simulink library "util_orbit_dynamics_lib"  (R2015b)
settings: Solver=VariableStepAuto  StartTime=0.0  StopTime=10.0  RelTol=1e-3
undefined symbols (not defined in the file or in its folder): central_body_gravity_mu, dt_perigee, ecc_anom, mean_anom, true_anom
libraries: util_orbit_dynamics_lib x15, util_common_lib x8, simulink_extras x2
settings Model: Creator=Mark Agbayani  LastModifiedBy=Mark Agbayani

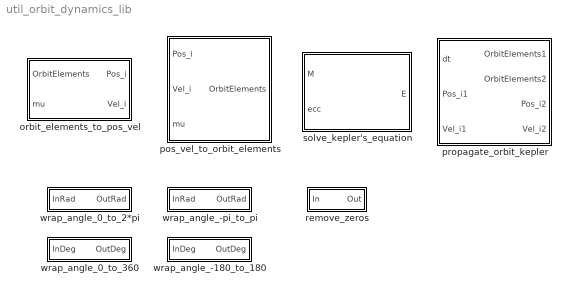
== system util_orbit_dynamics_lib ==
  orbit_elements_to_pos_vel : Subsystem
  pos_vel_to_orbit_elements : Subsystem
  propagate_orbit_kepler : Subsystem
  remove_zeros : Subsystem
  solve_kepler's_equation : Subsystem
  wrap_angle_-180_to_180 : Subsystem
      mask Display:
      | text(.5,.5,'-180< ang <+180', ...
      | 	'HorizontalAlignment','Center',...
      | 	'VerticalAlignment','middle')
  wrap_angle_-pi_to_pi : Subsystem
      mask Display:
      | text(.5,.5,'-pi < ang < +pi', ...
      | 	'HorizontalAlignment','Center',...
      | 	'VerticalAlignment','middle')
  wrap_angle_0_to_2*pi : Subsystem
      mask Display:
      | text(0.5,0.5,'0 < ang < 2*pi', ...
      | 	'HorizontalAlignment','Center',...
      | 	'VerticalAlignment','middle')
  wrap_angle_0_to_360 : Subsystem
      mask Display:
      | text(0.5,0.5,'0 < ang < 360', ...
      | 	'HorizontalAlignment','Center',...
      | 	'VerticalAlignment','middle')

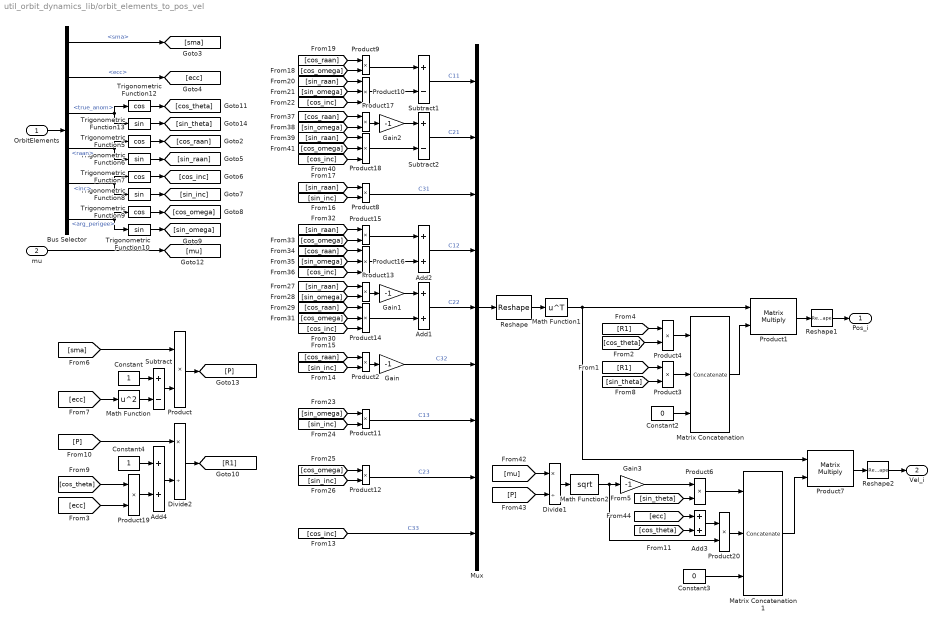
== system util_orbit_dynamics_lib/orbit_elements_to_pos_vel ==
  OrbitElements : Inport
  mu : Inport  Port=2
  Add{1..4} (4 alike) : Sum
  Bus Selector : BusSelector  OutputSignals=sma,ecc,true_anom,raan,inc,arg_perigee
  Constant : Constant
  Constant2 : Constant  Value=0
  Constant3 : Constant  Value=0
  Constant4 : Constant
  Divide1 : Product  Inputs=*/
  Divide2 : Product  Inputs=*/
  Gain{,1..3} (4 alike) : Gain  Gain=-1
  Math Function : Math  Operator=square  SaturateOnIntegerOverflow=on
  Math Function1 : Math  Operator=transpose  SaturateOnIntegerOverflow=on
  Math Function2 : Math  Operator=sqrt  SaturateOnIntegerOverflow=on
  Matrix Concatenation : Concatenate  NumInputs=3  Mode=Multidimensional array
  Matrix Concatenation1 : Concatenate  NumInputs=3  Mode=Multidimensional array
  Mux : Mux  Inputs=9
  Product{,2..4,6,8..9,11..13,15,17,19..20} (14 alike) : Product  RndMeth=Zero
  Product1 : Product  Multiplication=Matrix(*)  RndMeth=Zero
  Product{10,14,16,18} (4 alike) : Product  Inputs=3  RndMeth=Zero
  Product7 : Product  Multiplication=Matrix(*)  RndMeth=Zero
  Reshape : Reshape  OutputDimensionality=Customize  OutputDimensions=[3,3]
  Reshape1 : Reshape
  Reshape2 : Reshape
  Subtract : Sum  Inputs=+-
  Subtract1 : Sum  Inputs=+-
  Subtract2 : Sum  Inputs=+-
  Trigonometric Function{6,8,10,13} (4 alike) : Trigonometry
  Trigonometric Function{5,7,9,12} (4 alike) : Trigonometry  Operator=cos
  Pos_i : Outport
  Vel_i : Outport  Port=2
  wires:
  Matrix Concatenation1/1 -> Product7/2
  mu/1 -> [mu]
  [ecc] -> Math Function/1
  Constant/1 -> Subtract/1
  Math Function/1 -> Subtract/2
  Subtract/1 -> Product/2
  [sma] -> Product/1
  Product/1 -> [P]
  [R1] -> Product4/1
  [cos_theta] -> Product4/2
  Product4/1 -> Matrix Concatenation/1
  Product3/1 -> Matrix Concatenation/2
  Constant2/1 -> Matrix Concatenation/3
  Product6/1 -> Matrix Concatenation1/1
  Constant3/1 -> Matrix Concatenation1/3
  Mux/1 -> Reshape/1
  Reshape/1 -> Math Function1/1
  Trigonometric Function5/1 -> [cos_raan]
  Trigonometric Function6/1 -> [sin_raan]
  Trigonometric Function7/1 -> [cos_inc]
  Trigonometric Function8/1 -> [sin_inc]
  Trigonometric Function9/1 -> [cos_omega]
  Trigonometric Function10/1 -> [sin_omega]
  [cos_inc] -> Mux/9  "C33"
  Gain/1 -> Mux/6  "C32"
  Product2/1 -> Gain/1
  [cos_raan] -> Product2/1
  [sin_inc] -> Product2/2
  [sin_raan] -> Product8/1
  [sin_inc] -> Product8/2
  Product8/1 -> Mux/3  "C31"
  Subtract1/1 -> Mux/1  "C11"
  [cos_raan] -> Product9/1
  [cos_omega] -> Product9/2
  Product9/1 -> Subtract1/1
  Product10/1 -> Subtract1/2
  [sin_raan] -> Product10/1
  [sin_omega] -> Product10/2
  [cos_inc] -> Product10/3
  Product11/1 -> Mux/7  "C13"
  [sin_omega] -> Product11/1
  [sin_inc] -> Product11/2
  Math Function1/1 -> Product1/1, Product7/1
  [cos_omega] -> Product12/1
  [sin_inc] -> Product12/2
  Product12/1 -> Mux/8  "C23"
  [sin_raan] -> Product13/1
  [sin_omega] -> Product13/2
  Product13/1 -> Gain1/1
  Gain1/1 -> Add1/1
  [cos_raan] -> Product14/1
  [cos_omega] -> Product14/2
  [cos_inc] -> Product14/3
  Product14/1 -> Add1/2
  Add1/1 -> Mux/5  "C22"
  Subtract2/1 -> Mux/2  "C21"
  Add2/1 -> Mux/4  "C12"
  [sin_raan] -> Product15/1
  [cos_omega] -> Product15/2
  Product15/1 -> Add2/1
  Product16/1 -> Add2/2
  [cos_raan] -> Product16/1
  [sin_omega] -> Product16/2
  [cos_inc] -> Product16/3
  [cos_raan] -> Product17/1
  [sin_omega] -> Product17/2
  Product17/1 -> Gain2/1
  Gain2/1 -> Subtract2/1
  [sin_raan] -> Product18/1
  [cos_omega] -> Product18/2
  [cos_inc] -> Product18/3
  Product18/1 -> Subtract2/2
  [mu] -> Divide1/1
  [P] -> Divide1/2
  Divide1/1 -> Math Function2/1
  Math Function2/1 -> Gain3/1, Product20/2
  [sin_theta] -> Product6/2
  [cos_theta] -> Add3/2
  Gain3/1 -> Product6/1
  [ecc] -> Add3/1
  Add3/1 -> Product20/1
  Product20/1 -> Matrix Concatenation1/2
  Matrix Concatenation/1 -> Product1/2
  [P] -> Divide2/1
  Add4/1 -> Divide2/2
  Constant4/1 -> Add4/1
  [cos_theta] -> Product19/1
  Product19/1 -> Add4/2
  [ecc] -> Product19/2
  Divide2/1 -> [R1]
  Trigonometric Function12/1 -> [cos_theta]
  Trigonometric Function13/1 -> [sin_theta]
  [R1] -> Product3/1
  [sin_theta] -> Product3/2
  OrbitElements/1 -> Bus Selector/1
  Bus Selector/1 -> [sma]  "<sma>"
  Bus Selector/2 -> [ecc]  "<ecc>"
  Bus Selector/3 -> Trigonometric Function12/1, Trigonometric Function13/1  "<true_anom>"
  Bus Selector/4 -> Trigonometric Function5/1, Trigonometric Function6/1  "<raan>"
  Bus Selector/5 -> Trigonometric Function8/1, Trigonometric Function7/1  "<inc>"
  Bus Selector/6 -> Trigonometric Function9/1, Trigonometric Function10/1  "<arg_perigee>"
  Product1/1 -> Reshape1/1
  Product7/1 -> Reshape2/1
  Reshape1/1 -> Pos_i/1
  Reshape2/1 -> Vel_i/1

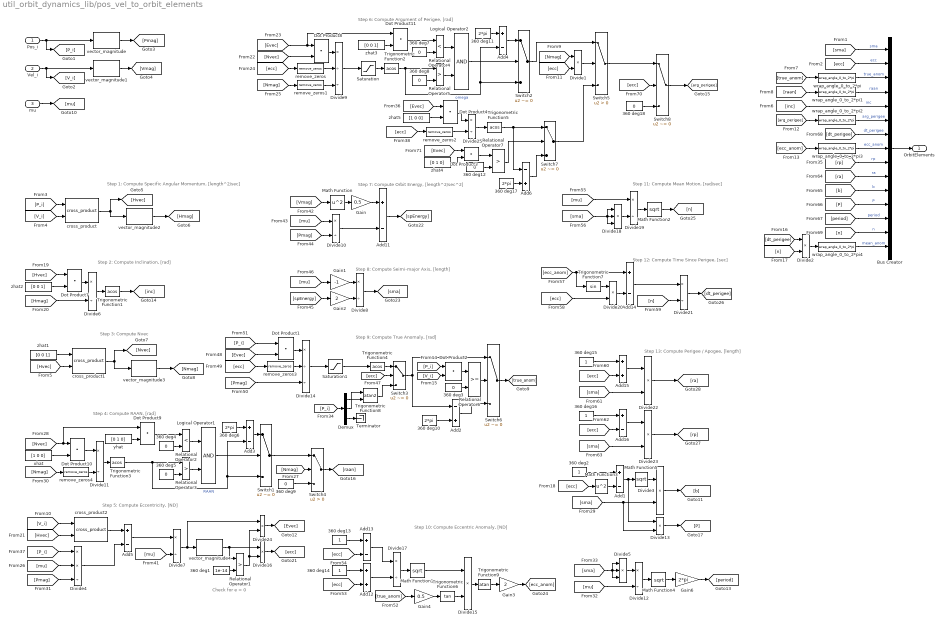
== system util_orbit_dynamics_lib/pos_vel_to_orbit_elements ==
  note: Step 1: Compute Specific Angular Momentum, [length^2/sec]
  note: Step 2: Compute Inclination, [rad]
  note: Step 3: Compute Nvec
  note: Step 4: Compute RAAN, [rad]
  note: Step 5: Compute Eccentricity, [ND]
  note: Step 6: Compute Argument of Perigee, [rad]
  note: Step 7: Compute Orbit Energy, [length^2/sec^2]
  note: Step 8: Compute Seimi-major Axis, [length]
  note: Step 9: Compute True Anomaly, [rad]
  note: Step 10: Compute Eccentric Anomaly, [ND]
  note: Step 11: Compute Mean Motion, [rad/sec]
  note: Step 12: Compute Time Since Perigee, [sec]
  note: Step 13: Compute Perigee / Apogee, [length]
  note: Check for e = 0
  Pos_i : Inport
  Vel_i : Inport  Port=2
  mu : Inport  Port=3
  360 deg1 : Constant  Value=1e-14
  360 deg{6,10..11,17} (4 alike) : Constant  Value=2*pi
  360 deg{3..5,7..9,12,18} (8 alike) : Constant  Value=0
  360 deg{2,13..16} (5 alike) : Constant
  Add{1,3..5,11,13..14,16} (8 alike) : Sum  Inputs=+-
  Add12 : Sum
  Add15 : Sum
  Add2 : Sum  Inputs=-+
  Add6 : Sum  Inputs=-+
  Bus Creator : BusCreator  Inputs=15
  Demux : Demux  Outputs=3
  Divide{1..3,13,15..16,20,22..24} (10 alike) : Product  Inputs=**
  Divide{6..8,10..12,17,19,21,25} (10 alike) : Product  Inputs=*/
  Divide14 : Product  Inputs=*//
  Divide18 : Product  Inputs=***
  Divide4 : Product  Inputs=**/
  Divide5 : Product  Inputs=***
  Divide9 : Product  Inputs=*//
  Dot Product{1..4,7..11} (9 alike) : DotProduct  InputSameDT=on  OutDataTypeStr=Inherit: Inherit via internal rule
  Gain : Gain  Gain=0.5
  Gain1 : Gain  Gain=-1
  Gain2 : Gain  Gain=2
  Gain3 : Gain  Gain=2
  Gain4 : Gain  Gain=0.5
  Gain6 : Gain  Gain=2*pi
  Logical Operator1 : Logic  AllPortsSameDT=off  OutDataTypeStr=float('double')
  Logical Operator2 : Logic  AllPortsSameDT=off  OutDataTypeStr=float('double')
  Math Function : Math  Operator=square  SaturateOnIntegerOverflow=on
  Math Function{1..2,4..5} (4 alike) : Math  Operator=sqrt  SaturateOnIntegerOverflow=on
  Math Function3 : Math  Operator=square  SaturateOnIntegerOverflow=on
  Relational Operator1 : RelationalOperator  Operator=>  OutDataTypeStr=float('double')
  Relational Operator2 : RelationalOperator  Operator=<  OutDataTypeStr=boolean
  Relational Operator3 : RelationalOperator  Operator=>  OutDataTypeStr=boolean
  Relational Operator4 : RelationalOperator  Operator=<  OutDataTypeStr=boolean
  Relational Operator5 : RelationalOperator  Operator=>  OutDataTypeStr=boolean
  Relational Operator6 : RelationalOperator  OutDataTypeStr=float('double')
  Relational Operator7 : RelationalOperator  Operator=>  OutDataTypeStr=float('double')
  Saturation : Saturate  UpperLimit=1  LowerLimit=-1
  Saturation1 : Saturate  UpperLimit=1  LowerLimit=-1
  Switch{1..3,6..8} (6 alike) : Switch  Criteria=u2 ~= 0
  Switch4 : Switch  Criteria=u2 > Threshold
  Switch5 : Switch  Criteria=u2 > Threshold
  Terminator : Terminator
  Trigonometric Function{1..5} (5 alike) : Trigonometry  Operator=acos
  Trigonometric Function6 : Trigonometry  Operator=tan
  Trigonometric Function7 : Trigonometry
  Trigonometric Function8 : Trigonometry  Operator=atan2
  Trigonometric Function9 : Trigonometry  Operator=atan
  cross_product : util_common_lib/cross_product  SystemSampleTime=-1
  cross_product1 : util_common_lib/cross_product  SystemSampleTime=-1
  cross_product2 : util_common_lib/cross_product  SystemSampleTime=-1
  remove_zeros{,1..4} (5 alike) : util_orbit_dynamics_lib/remove_zeros  SystemSampleTime=-1
  vector_magnitude{,1..4} (5 alike) : util_common_lib/vector_magnitude  SystemSampleTime=-1
  wrap_angle_0_to_2*pi{,1..4} (5 alike) : util_orbit_dynamics_lib/wrap_angle_0_to_2*pi  SystemSampleTime=-1
  xhat : Constant  Value=[1 0 0]
  yhat : Constant  Value=[0 1 0]
  zhat1 : Constant  Value=[0 0 1]
  zhat2 : Constant  Value=[0 0 1]
  zhat3 : Constant  Value=[0 0 1]
  zhat4 : Constant  Value=[0 1 0]
  zhat5 : Constant  Value=[1 0 0]
  OrbitElements : Outport
  wires:
  wrap_angle_0_to_2*pi4/1 -> Bus Creator/15  "mean_anom"
  [n] -> Bus Creator/14  "n"
  [period] -> Bus Creator/13  "period"
  [P] -> Bus Creator/12  "P"
  [b] -> Bus Creator/11  "b"
  [ra] -> Bus Creator/10  "ra"
  [rp] -> Bus Creator/9  "rp"
  wrap_angle_0_to_2*pi3/1 -> Bus Creator/8  "ecc_anom"
  [dt_perigee] -> Bus Creator/7  "dt_perigee"
  [sma] -> Divide23/2
  [ecc] -> Add16/2
  Add16/1 -> Divide23/1
  360 deg16/1 -> Add16/1
  [sma] -> Divide22/2
  [ecc] -> Add15/2
  Add15/1 -> Divide22/1
  360 deg15/1 -> Add15/1
  Divide21/1 -> [dt_perigee]
  [n] -> Divide21/2
  Add14/1 -> Divide21/1
  Divide20/1 -> Add14/2
  [ecc] -> Divide20/2
  Trigonometric Function7/1 -> Divide20/1
  [ecc_anom] -> Trigonometric Function7/1, Add14/1
  Math Function2/1 -> [n]
  Divide19/1 -> Math Function2/1
  [sma] -> Divide18/3, Divide18/2, Divide18/1
  Divide18/1 -> Divide19/2
  [mu] -> Divide19/1
  Add12/1 -> Divide17/2
  Add13/1 -> Divide17/1
  [ecc] -> Add13/2
  360 deg13/1 -> Add13/1
  [ecc] -> Add12/2
  360 deg14/1 -> Add12/1
  Divide17/1 -> Math Function1/1
  Gain4/1 -> Trigonometric Function6/1
  [true_anom] -> Gain4/1
  Trigonometric Function6/1 -> Divide15/2
  Math Function1/1 -> Divide15/1
  Divide15/1 -> Trigonometric Function9/1
  Gain3/1 -> [ecc_anom]
  Dot Product1/1 -> Divide14/1
  [Pmag] -> Divide14/3
  [Evec] -> Dot Product1/2
  [P_i] -> Dot Product1/1
  Trigonometric Function4/1 -> Switch3/1
  [ecc] -> Switch3/2
  Divide8/1 -> [sma]
  Gain1/1 -> Divide8/1
  Gain2/1 -> Divide8/2
  [spEnergy] -> Gain2/1
  [mu] -> Gain1/1
  Add11/1 -> [spEnergy]
  Math Function/1 -> Gain/1
  Gain/1 -> Add11/1
  Divide10/1 -> Add11/2
  [Pmag] -> Divide10/2
  [mu] -> Divide10/1
  [Vmag] -> Math Function/1
  vector_magnitude4/1 -> Relational Operator1/1, Divide16/1
  Divide7/1 -> vector_magnitude4/1, Divide24/1
  [mu] -> Divide7/2
  Add5/1 -> Divide7/1
  Divide4/1 -> Add5/2
  [Pmag] -> Divide4/3
  [mu] -> Divide4/2
  [P_i] -> Divide4/1
  [Hvec] -> cross_product2/2
  [V_i] -> cross_product2/1
  cross_product2/1 -> Add5/1
  Dot Product9/1 -> Relational Operator2/1
  Add3/1 -> Switch1/1
  Logical Operator1/1 -> Switch1/2
  360 deg6/1 -> Add3/1
  Relational Operator3/1 -> Logical Operator1/2
  Relational Operator2/1 -> Logical Operator1/1
  360 deg5/1 -> Relational Operator3/2
  360 deg4/1 -> Relational Operator2/2
  yhat/1 -> Dot Product9/2
  Bus Creator/1 -> OrbitElements/1
  wrap_angle_0_to_2*pi2/1 -> Bus Creator/6  "arg_perigee"
  [inc] -> Bus Creator/5  "inc"
  wrap_angle_0_to_2*pi1/1 -> Bus Creator/4  "raan"
  wrap_angle_0_to_2*pi/1 -> Bus Creator/3  "true_anom"
  [ecc] -> Bus Creator/2  "ecc"
  [sma] -> Bus Creator/1  "sma"
  [Nvec] -> Dot Product9/1, Dot Product10/1
  [Nmag] -> remove_zeros4/1
  Trigonometric Function3/1 -> Switch1/3, Add3/2, Relational Operator3/1  "RAAN"
  Divide11/1 -> Trigonometric Function3/1
  Dot Product10/1 -> Divide11/1
  xhat/1 -> Dot Product10/2
  Divide6/1 -> Trigonometric Function1/1
  Trigonometric Function1/1 -> [inc]
  Dot Product7/1 -> Divide6/1
  [Hmag] -> Divide6/2
  [Hvec] -> Dot Product7/1
  zhat2/1 -> Dot Product7/2
  zhat1/1 -> cross_product1/1
  [Hvec] -> cross_product1/2
  cross_product1/1 -> vector_magnitude3/1, [Nvec]
  vector_magnitude3/1 -> [Nmag]
  cross_product/1 -> vector_magnitude2/1, [Hvec]
  vector_magnitude2/1 -> [Hmag]
  [V_i] -> cross_product/2
  [P_i] -> cross_product/1
  Vel_i/1 -> vector_magnitude1/1, [V_i]
  vector_magnitude/1 -> [Pmag]
  vector_magnitude1/1 -> [Vmag]
  Pos_i/1 -> vector_magnitude/1, [P_i]
  [true_anom] -> wrap_angle_0_to_2*pi/1
  [raan] -> wrap_angle_0_to_2*pi1/1
  [arg_perigee] -> wrap_angle_0_to_2*pi2/1
  [ecc_anom] -> wrap_angle_0_to_2*pi3/1
  mu/1 -> [mu]
  [Nmag] -> Switch4/2
  360 deg9/1 -> Switch4/3
  Switch4/1 -> [raan]
  Switch1/1 -> Switch4/1
  Divide14/1 -> Saturation1/1
  [Evec] -> Dot Product11/1, Dot Product8/1
  Dot Product11/1 -> Relational Operator4/1
  Add4/1 -> Switch2/1
  Logical Operator2/1 -> Switch2/2
  360 deg11/1 -> Add4/1
  Relational Operator5/1 -> Logical Operator2/2
  Relational Operator4/1 -> Logical Operator2/1
  360 deg8/1 -> Relational Operator5/2
  360 deg7/1 -> Relational Operator4/2
  zhat3/1 -> Dot Product11/2
  Trigonometric Function2/1 -> Switch2/3, Add4/2, Relational Operator5/1  "omega"
  Divide9/1 -> Saturation/1
  Dot Product8/1 -> Divide9/1
  [Nmag] -> remove_zeros1/1
  [ecc] -> remove_zeros/1
  [Nvec] -> Dot Product8/2
  [Nmag] -> Divide1/1
  [ecc] -> Divide1/2
  Divide1/1 -> Switch5/2
  Switch2/1 -> Switch5/1
  Switch6/1 -> [true_anom]
  Switch3/1 -> Switch6/1, Add2/1
  [P_i] -> Dot Product2/1
  [V_i] -> Dot Product2/2
  [dt_perigee] -> Divide2/1
  [n] -> Divide2/2
  Divide2/1 -> wrap_angle_0_to_2*pi4/1
  [sma] -> Divide3/2, Divide13/2
  [ecc] -> Math Function3/1
  Add1/1 -> Math Function5/1, Divide13/1
  360 deg2/1 -> Add1/1
  Math Function3/1 -> Add1/2
  Divide3/1 -> [b]
  Divide12/1 -> Math Function4/1
  [sma] -> Divide5/2, Divide5/3, Divide5/1
  Divide5/1 -> Divide12/1
  [mu] -> Divide12/2
  Math Function4/1 -> Gain6/1
  Gain6/1 -> [period]
  Math Function5/1 -> Divide3/1
  Divide13/1 -> [P]
  Divide23/1 -> [rp]
  Divide22/1 -> [ra]
  [P_i] -> Demux/1
  Demux/3 -> Terminator/1
  Demux/1 -> Trigonometric Function8/2
  Demux/2 -> Trigonometric Function8/1
  Trigonometric Function8/1 -> Switch3/3
  360 deg1/1 -> Relational Operator1/2
  Relational Operator1/1 -> Divide16/2, Divide24/2
  Divide16/1 -> [ecc]
  Divide24/1 -> [Evec]
  Dot Product2/1 -> Relational Operator6/1
  360 deg3/1 -> Relational Operator6/2
  Relational Operator6/1 -> Switch6/2
  remove_zeros1/1 -> Divide9/3
  remove_zeros/1 -> Divide9/2
  remove_zeros4/1 -> Divide11/2
  Trigonometric Function9/1 -> Gain3/1
  zhat5/1 -> Dot Product4/2
  [Evec] -> Dot Product4/1
  Dot Product4/1 -> Divide25/1
  [ecc] -> remove_zeros2/1
  remove_zeros2/1 -> Divide25/2
  Divide25/1 -> Trigonometric Function5/1
  [ecc] -> remove_zeros3/1
  remove_zeros3/1 -> Divide14/2
  360 deg10/1 -> Add2/2
  Add2/1 -> Switch6/3
  Saturation1/1 -> Trigonometric Function4/1
  Saturation/1 -> Trigonometric Function2/1
  Trigonometric Function5/1 -> Switch7/1, Add6/1
  360 deg12/1 -> Relational Operator7/2
  Dot Product3/1 -> Relational Operator7/1
  Relational Operator7/1 -> Switch7/2
  360 deg17/1 -> Add6/2
  Add6/1 -> Switch7/3
  Switch7/1 -> Switch5/3
  zhat4/1 -> Dot Product3/2
  [Evec] -> Dot Product3/1
  Switch5/1 -> Switch8/1
  [ecc] -> Switch8/2
  360 deg18/1 -> Switch8/3
  Switch8/1 -> [arg_perigee]

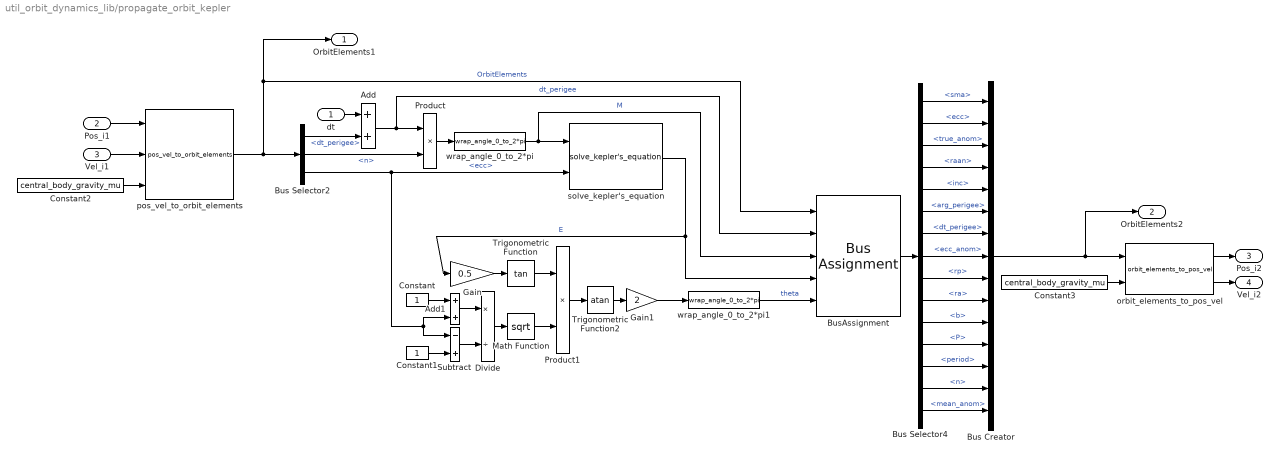
== system util_orbit_dynamics_lib/propagate_orbit_kepler ==
  dt : Inport
  Pos_i1 : Inport  Port=2
  Vel_i1 : Inport  Port=3
  Add : Sum
  Add1 : Sum
  Bus Creator : BusCreator  Inputs=15
  Bus Selector2 : BusSelector  OutputSignals=dt_perigee,n,ecc
  Bus Selector4 : BusSelector  OutputSignals=sma,ecc,true_anom,raan,inc,arg_perigee,dt_perigee,ecc_anom,rp,ra,b,P,period,n,mean_anom
  BusAssignment : BusAssignment  AssignedSignals=dt_perigee,mean_anom,ecc_anom,true_anom
  Constant : Constant
  Constant1 : Constant
  Constant2 : Constant  Value=central_body_gravity_mu
  Constant3 : Constant  Value=central_body_gravity_mu
  Divide : Product  Inputs=*/
  Gain : Gain  Gain=0.5
  Gain1 : Gain  Gain=2
  Math Function : Math  Operator=sqrt  SaturateOnIntegerOverflow=on
  Product : Product  RndMeth=Zero
  Product1 : Product  RndMeth=Zero
  Subtract : Sum  Inputs=-+
  Trigonometric Function : Trigonometry  Operator=tan
  Trigonometric Function2 : Trigonometry  Operator=atan
  orbit_elements_to_pos_vel : util_orbit_dynamics_lib/orbit_elements_to_pos_vel
  pos_vel_to_orbit_elements : util_orbit_dynamics_lib/pos_vel_to_orbit_elements
  solve_kepler's_equation : util_orbit_dynamics_lib/solve_kepler's_equation
  wrap_angle_0_to_2*pi : util_orbit_dynamics_lib/wrap_angle_0_to_2*pi  SystemSampleTime=-1
  wrap_angle_0_to_2*pi1 : util_orbit_dynamics_lib/wrap_angle_0_to_2*pi  SystemSampleTime=-1
  OrbitElements1 : Outport
  OrbitElements2 : Outport  Port=2
  Pos_i2 : Outport  Port=3
  Vel_i2 : Outport  Port=4
  wires:
  pos_vel_to_orbit_elements/1 -> Bus Selector2/1, BusAssignment/1, OrbitElements1/1  "OrbitElements"
  Pos_i1/1 -> pos_vel_to_orbit_elements/1
  Vel_i1/1 -> pos_vel_to_orbit_elements/2
  orbit_elements_to_pos_vel/1 -> Pos_i2/1
  orbit_elements_to_pos_vel/2 -> Vel_i2/1
  Bus Selector2/1 -> Add/2  "<dt_perigee>"
  dt/1 -> Add/1
  Bus Selector2/2 -> Product/2  "<n>"
  Add/1 -> Product/1, BusAssignment/2  "dt_perigee"
  Product/1 -> wrap_angle_0_to_2*pi/1
  wrap_angle_0_to_2*pi/1 -> solve_kepler's_equation/1, BusAssignment/3  "M"
  Bus Selector2/3 -> solve_kepler's_equation/2, Add1/2, Subtract/1  "<ecc>"
  solve_kepler's_equation/1 -> BusAssignment/4, Gain/1  "E"
  Math Function/1 -> Product1/2
  Divide/1 -> Math Function/1
  Add1/1 -> Divide/1
  Constant/1 -> Add1/1
  Subtract/1 -> Divide/2
  Constant1/1 -> Subtract/2
  Gain/1 -> Trigonometric Function/1
  Trigonometric Function/1 -> Product1/1
  Product1/1 -> Trigonometric Function2/1
  Trigonometric Function2/1 -> Gain1/1
  Gain1/1 -> wrap_angle_0_to_2*pi1/1
  Constant3/1 -> orbit_elements_to_pos_vel/2
  Constant2/1 -> pos_vel_to_orbit_elements/3
  wrap_angle_0_to_2*pi1/1 -> BusAssignment/5  "theta"
  BusAssignment/1 -> Bus Selector4/1
  Bus Selector4/1 -> Bus Creator/1  "<sma>"
  Bus Selector4/2 -> Bus Creator/2  "<ecc>"
  Bus Selector4/3 -> Bus Creator/3  "<true_anom>"
  Bus Selector4/4 -> Bus Creator/4  "<raan>"
  Bus Selector4/5 -> Bus Creator/5  "<inc>"
  Bus Selector4/6 -> Bus Creator/6  "<arg_perigee>"
  Bus Selector4/7 -> Bus Creator/7  "<dt_perigee>"
  Bus Selector4/8 -> Bus Creator/8  "<ecc_anom>"
  Bus Selector4/9 -> Bus Creator/9  "<rp>"
  Bus Selector4/10 -> Bus Creator/10  "<ra>"
  Bus Selector4/11 -> Bus Creator/11  "<b>"
  Bus Selector4/12 -> Bus Creator/12  "<P>"
  Bus Selector4/13 -> Bus Creator/13  "<period>"
  Bus Selector4/14 -> Bus Creator/14  "<n>"
  Bus Selector4/15 -> Bus Creator/15  "<mean_anom>"
  Bus Creator/1 -> orbit_elements_to_pos_vel/1, OrbitElements2/1

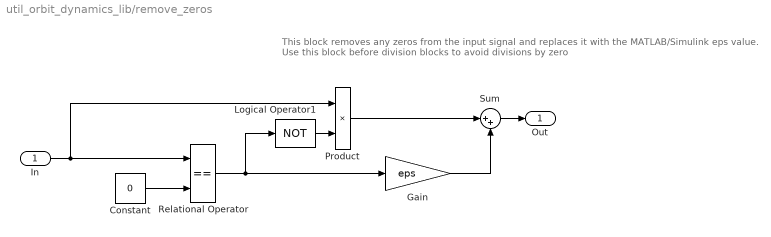
== system util_orbit_dynamics_lib/remove_zeros ==
  note: This block removes any zeros from the input signal and replaces
      | it with the MATLAB/Simulink eps value.
      | Use this block before division blocks to avoid divisions by zero
  In : Inport
  Constant : Constant  Value=0
  Gain : Gain  Gain=eps
  Logical Operator1 : Logic  Operator=NOT  AllPortsSameDT=off  OutDataTypeStr=float('double')
  Product : Product  RndMeth=Zero
  Relational Operator : RelationalOperator  Operator===  OutDataTypeStr=float('double')
  Sum : Sum  Inputs=|++
  Out : Outport
  wires:
  In/1 -> Product/1, Relational Operator/1
  Relational Operator/1 -> Gain/1, Logical Operator1/1
  Gain/1 -> Sum/2
  Logical Operator1/1 -> Product/2
  Product/1 -> Sum/1
  Sum/1 -> Out/1
  Constant/1 -> Relational Operator/2

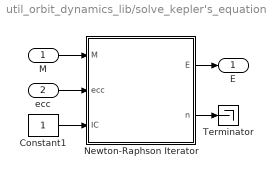
== system util_orbit_dynamics_lib/solve_kepler's_equation ==
  M : Inport
  ecc : Inport  Port=2
  Constant1 : Constant
  Newton-Raphson Iterator : Subsystem
  Terminator : Terminator
  E : Outport
  wires:
  ecc/1 -> Newton-Raphson Iterator/2(ecc)
  Constant1/1 -> Newton-Raphson Iterator/3(IC)
  Newton-Raphson Iterator/2(n) -> Terminator/1
  M/1 -> Newton-Raphson Iterator/1(M)
  Newton-Raphson Iterator/1(E) -> E/1

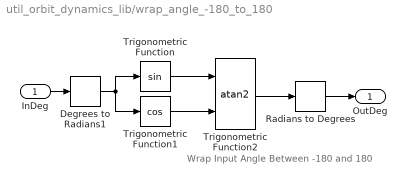
== system util_orbit_dynamics_lib/wrap_angle_-180_to_180 ==
  note: Wrap Input Angle Between -180 and 180
  InDeg : Inport
  Degrees to Radians1 : simulink_extras/Transformations/Degrees to Radians
  Radians to Degrees : simulink_extras/Transformations/Radians to Degrees
  Trigonometric Function : Trigonometry
  Trigonometric Function1 : Trigonometry  Operator=cos
  Trigonometric Function2 : Trigonometry  Operator=atan2
  OutDeg : Outport
  wires:
  Degrees to Radians1/1 -> Trigonometric Function/1, Trigonometric Function1/1
  Radians to Degrees/1 -> OutDeg/1
  Trigonometric Function/1 -> Trigonometric Function2/1
  Trigonometric Function1/1 -> Trigonometric Function2/2
  InDeg/1 -> Degrees to Radians1/1
  Trigonometric Function2/1 -> Radians to Degrees/1

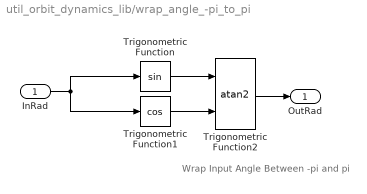
== system util_orbit_dynamics_lib/wrap_angle_-pi_to_pi ==
  note: Wrap Input Angle Between -pi and pi
  InRad : Inport
  Trigonometric Function : Trigonometry
  Trigonometric Function1 : Trigonometry  Operator=cos
  Trigonometric Function2 : Trigonometry  Operator=atan2
  OutRad : Outport
  wires:
  Trigonometric Function2/1 -> OutRad/1
  InRad/1 -> Trigonometric Function1/1, Trigonometric Function/1
  Trigonometric Function1/1 -> Trigonometric Function2/2
  Trigonometric Function/1 -> Trigonometric Function2/1

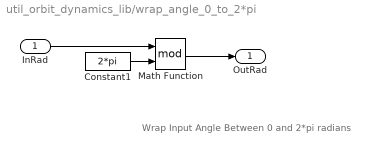
== system util_orbit_dynamics_lib/wrap_angle_0_to_2*pi ==
  note: Wrap Input Angle Between 0 and 2*pi radians
  InRad : Inport
  Constant1 : Constant  Value=2*pi
  Math Function : Math  Operator=mod  SaturateOnIntegerOverflow=on
  OutRad : Outport
  wires:
  InRad/1 -> Math Function/1
  Constant1/1 -> Math Function/2
  Math Function/1 -> OutRad/1

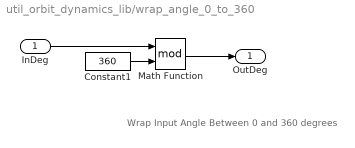
== system util_orbit_dynamics_lib/wrap_angle_0_to_360 ==
  note: Wrap Input Angle Between 0 and 360 degrees
  InDeg : Inport
  Constant1 : Constant  Value=360
  Math Function : Math  Operator=mod  SaturateOnIntegerOverflow=on
  OutDeg : Outport
  wires:
  Math Function/1 -> OutDeg/1
  Constant1/1 -> Math Function/2
  InDeg/1 -> Math Function/1

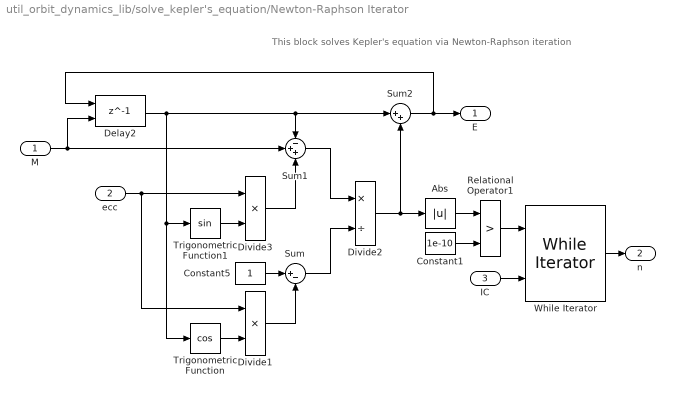
== system util_orbit_dynamics_lib/solve_kepler's_equation/Newton-Raphson Iterator ==
  note: This block solves Kepler's equation via Newton-Raphson iteration
  M : Inport
  ecc : Inport  Port=2
  IC : Inport  Port=3
  Abs : Abs
  Constant1 : Constant  Value=1e-10
  Constant5 : Constant
  Delay2 : Delay  DelayLength=1  InitialConditionSource=Input port
      settings: InputPortMap=u0,p4
  Divide1 : Product  Inputs=**
  Divide2 : Product  Inputs=*/
  Divide3 : Product  Inputs=**
  Relational Operator1 : RelationalOperator  Operator=>  OutDataTypeStr=boolean
  Sum : Sum  Inputs=|+-
  Sum1 : Sum  Inputs=-++
  Sum2 : Sum  Inputs=|++
  Trigonometric Function : Trigonometry  Operator=cos
  Trigonometric Function1 : Trigonometry
  While Iterator : WhileIterator  MaxIters=20  ResetStates=reset  ShowIterationPort=on  OutputDataType=int8
  E : Outport
  n : Outport  Port=2
  wires:
  IC/1 -> While Iterator/2
  Sum/1 -> Divide2/2
  Constant5/1 -> Sum/1
  Trigonometric Function/1 -> Divide1/2
  Divide1/1 -> Sum/2
  Trigonometric Function1/1 -> Divide3/2
  Sum1/1 -> Divide2/1
  Divide2/1 -> Abs/1, Sum2/2
  ecc/1 -> Divide1/1, Divide3/1
  Constant1/1 -> Relational Operator1/2
  Relational Operator1/1 -> While Iterator/1
  Abs/1 -> Relational Operator1/1
  Delay2/1 -> Trigonometric Function1/1, Trigonometric Function/1, Sum1/1, Sum2/1
  Divide3/1 -> Sum1/3
  Sum2/1 -> E/1, Delay2/1
  M/1 -> Delay2/2, Sum1/2
  While Iterator/1 -> n/1
